simulink model "real_timeID"  (R2024b)
settings: Solver=VariableStepAuto  StartTime=0.0  StopTime=40  RelTol=1e-3
values from neighbouring files (symbols this model uses):
  wn = 1    [real_timeID.m]    (also in real_timeID_script.m; realtime_ID_control.m; sim_real_timeID_script.m)
  xi = 0.3    [real_timeID_script.m]    (also in sim_real_timeID_script.m)
undefined symbols (not defined in the file or in its folder): s
libraries: fod x1
settings Model: Creator=r7fon  LastModifiedBy=r7fon

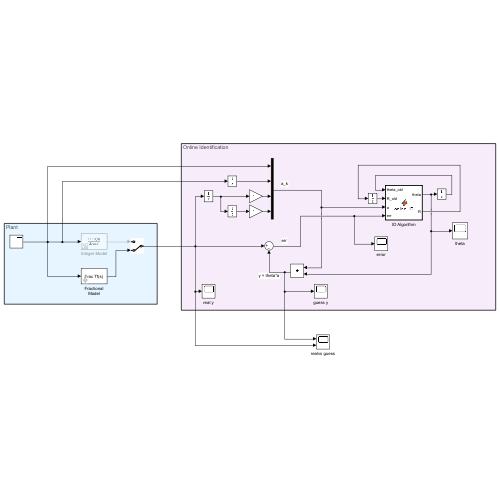
[thumbnail: Simulink's stored preview of the top-level diagram]
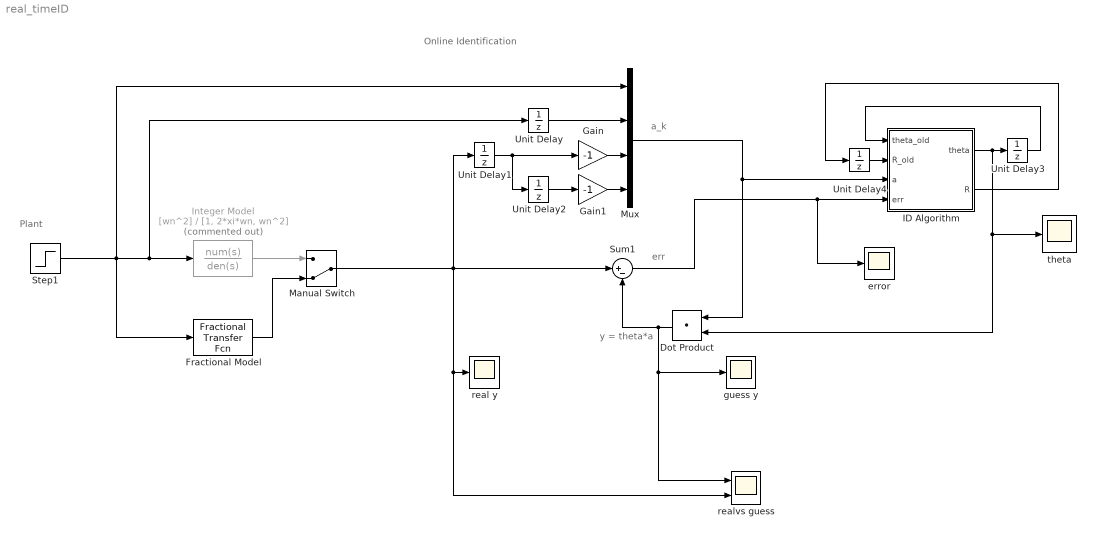
== system real_timeID ==
  note: Online Identification
  note: Plant
  note: a_k
  note: err
  note: y = theta*a
  Dot Product : DotProduct  OutDataTypeStr=Inherit: Inherit via internal rule
  Fractional Model : fod/Fractional Transfer Fcn  Tag=Fractional Transfer Fcn  Description=Fractional LTI system transfer function  zeroPoly=1  polePoly=1*s^2.2 + 4*s^1.2 + 1  freqRange=[0.001, 1000]  approxNum=5  useRef=off
      settings: SourceProductName=FOMCON Toolbox
  Gain : Gain  Gain=-1
  Gain1 : Gain  Gain=-1
  ID Algorithm : MATLAB Function  TreatAsAtomicUnit=on
  Integer Model : TransferFcn  Commented=on  Numerator=[wn^2]  Denominator=[1, 2*xi*wn, wn^2]
  Manual Switch : ManualSwitch  CurrentSetting=0
  Mux : Mux
  Step1 : Step  Time=0  SampleTime=0
  Sum1 : Sum  Inputs=|+-
  Unit Delay : UnitDelay  SampleTime=-1  HasFrameUpgradeWarning=on
  Unit Delay1 : UnitDelay  SampleTime=-1  HasFrameUpgradeWarning=on
  Unit Delay2 : UnitDelay  SampleTime=-1  HasFrameUpgradeWarning=on
  Unit Delay3 : UnitDelay  InitialCondition=zeros(4, 1)  SampleTime=-1  HasFrameUpgradeWarning=on
  Unit Delay4 : UnitDelay  InitialCondition=eye(4)*0.1  SampleTime=-1  HasFrameUpgradeWarning=on
  error : Scope
  guess y : Scope
  real y : Scope
  realvs guess : Scope  NumInputPorts=2
  theta : Scope
  wires:
  Step1/1 -> Fractional Model/1, Unit Delay/1, Integer Model/1, Mux/1
  Manual Switch/1 -> realvs guess/2, real y/1, Unit Delay1/1, Sum1/1
  Sum1/1 -> error/1, ID Algorithm/4(err)
  Unit Delay/1 -> Mux/2
  Gain/1 -> Mux/3
  Unit Delay1/1 -> Gain/1, Unit Delay2/1
  Gain1/1 -> Mux/4
  Unit Delay2/1 -> Gain1/1
  Mux/1 -> Dot Product/1, ID Algorithm/3(a)
  Dot Product/1 -> guess y/1, realvs guess/1, Sum1/2
  ID Algorithm/2(R) -> Unit Delay4/1
  Unit Delay4/1 -> ID Algorithm/2(R_old)
  ID Algorithm/1(theta) -> Dot Product/2, theta/1, Unit Delay3/1
  Unit Delay3/1 -> ID Algorithm/1(theta_old)
  Integer Model/1 -> Manual Switch/1
  Fractional Model/1 -> Manual Switch/2

== matlab function real_timeID/ID Algorithm ==
  data: theta_old input; R_old input; a input; err input; theta output; R output
function [theta,R] = online_ID(theta_old, R_old, a, err)


% forgetting factor
alpha = 1;


R = R_old + alpha*(a*a');
theta = theta_old + alpha*(R\a)*err;
    

end
